simulink model "aircraft_6dof"  (R2025a)
settings: Solver=VariableStepAuto  StartTime=0.0  StopTime=sim_params.duration  FixedStep=0.01  RelTol=1e-8
values from neighbouring files (symbols this model uses):
  aero = evalin('base', 'aero')    [trim_solver.m]
  aircraft = evalin('base', 'aircraft')    [trim_solver.m]
  atmos = evalin('base', 'atmos')    [trim_solver.m]
  engine = evalin('base', 'engine')    [trim_solver.m]
undefined symbols (not defined in the file or in its folder): IC
libraries: aerolibasang x2, aerolibtransform2 x1, aerolibatmos2 x1
settings Model: Creator=lordf  LastModifiedBy=lordf
settings DataIOCC: ExternalInput=getinputstruct(op2)  InitialState=getstatestruct(op2)  LoadExternalInput=on  LoadInitialState=on

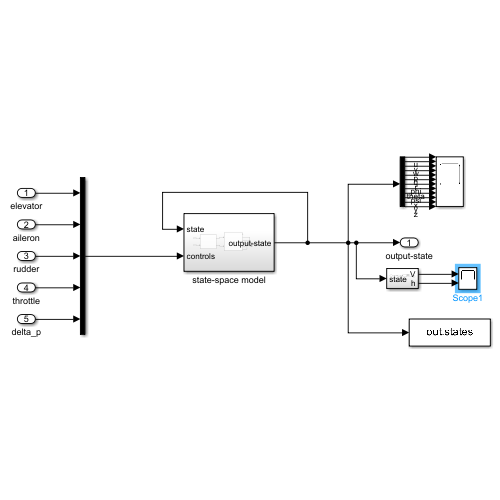
[thumbnail: Simulink's stored preview of the top-level diagram]
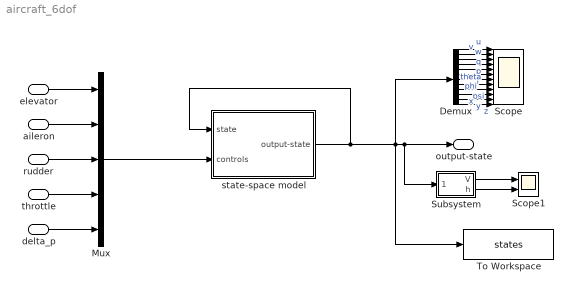
== system aircraft_6dof ==
  elevator : Inport
  aileron : Inport  Port=2
  rudder : Inport  Port=3
  throttle : Inport  Port=4
  delta_p : Inport  Port=5
  Demux : Demux  Outputs=12
  Mux : Mux  Inputs=5
  Scope : Scope  NumInputPorts=12
      settings: ActiveDisplayYMinimum=-1  ActiveDisplayYMaximum=1
  Scope1 : Scope  NumInputPorts=2
      settings: ActiveDisplayYMinimum=149.99795642842278  ActiveDisplayYMaximum=149.99795643262632
  Subsystem : Subsystem
  To Workspace : ToWorkspace  VariableName=states  SampleTime=-1
  state-space model : Subsystem
  output-state : Outport
  wires:
  state-space model/1(output-state) -> state-space model/1(state), Subsystem/1(state), output-state/1, Demux/1, To Workspace/1
  rudder/1 -> Mux/3
  aileron/1 -> Mux/2
  elevator/1 -> Mux/1
  throttle/1 -> Mux/4
  delta_p/1 -> Mux/5
  Mux/1 -> state-space model/2(controls)
  Demux/1 -> Scope/1  "u"
  Demux/2 -> Scope/2  "v"
  Demux/3 -> Scope/3  "w"
  Demux/4 -> Scope/4  "p"
  Demux/5 -> Scope/5  "q"
  Demux/6 -> Scope/6  "r"
  Demux/7 -> Scope/7  "phi"
  Demux/8 -> Scope/8  "theta"
  Demux/9 -> Scope/9  "psi"
  Demux/10 -> Scope/10  "x"
  Demux/11 -> Scope/11  "y"
  Demux/12 -> Scope/12  "z"
  Subsystem/2(h) -> Scope1/2
  Subsystem/1(V) -> Scope1/1

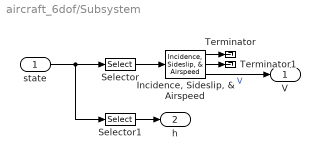
== system aircraft_6dof/Subsystem ==
  state : Inport
  "Incidence, Sideslip, & Airspeed" : aerolibasang/Incidence, Sideslip, & Airspeed
  Selector : Selector  InputPortWidth=12  IndexOptions=Index vector (dialog)  Indices=1:3  OutputSizes=1
  Selector1 : Selector  InputPortWidth=12  IndexOptions=Index vector (dialog)  Indices=12  OutputSizes=1
  Terminator : Terminator
  Terminator1 : Terminator
  V : Outport
  h : Outport  Port=2
  wires:
  Selector/1 -> "Incidence, Sideslip, & Airspeed"/1
  state/1 -> Selector1/1, Selector/1
  "Incidence, Sideslip, & Airspeed"/1 -> Terminator/1
  "Incidence, Sideslip, & Airspeed"/2 -> Terminator1/1
  "Incidence, Sideslip, & Airspeed"/3 -> V/1  "V"
  Selector1/1 -> h/1

== system aircraft_6dof/state-space model ==
  state : Inport
  controls : Inport  Port=2
  6DOF (Euler Angles) : EOM6DOFBodyEuler  xme_0=[IC.x IC.y IC.z]  Vm_0=[IC.u, IC.v, IC.w]  eul_0=[IC.phi IC.theta IC.psi]  pm_0=[IC.p IC.q IC.r]  mass_0=aircraft.mass  inertia=aircraft.I
  Forces and Moments : Subsystem
  Mux1 : Mux
  output-state : Outport
  wires:
  6DOF (Euler Angles)/3 -> Mux1/3  "attitude(earth)"
  6DOF (Euler Angles)/5 -> Mux1/1  "velocity(body)"
  Forces and Moments/2(M) -> 6DOF (Euler Angles)/2
  6DOF (Euler Angles)/2 -> Mux1/4  "Position(earth)"
  Forces and Moments/1(F) -> 6DOF (Euler Angles)/1
  6DOF (Euler Angles)/6 -> Mux1/2  "omega(body)"
  Mux1/1 -> output-state/1
  controls/1 -> Forces and Moments/2(controls)
  state/1 -> Forces and Moments/1(state)

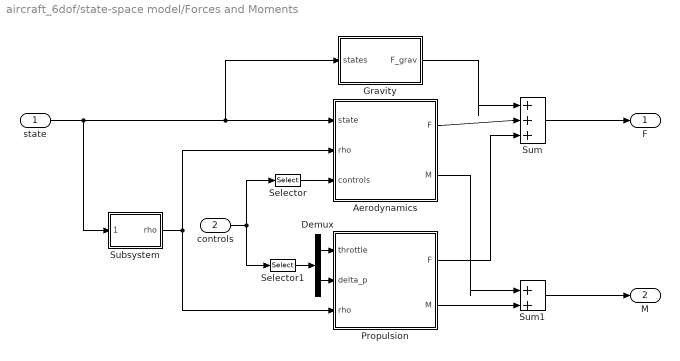
== system aircraft_6dof/state-space model/Forces and Moments ==
  state : Inport
  controls : Inport  Port=2
  Aerodynamics : Subsystem
  Demux : Demux  Outputs=2
  Gravity : Subsystem
  Propulsion : Subsystem
  Selector : Selector  InputPortWidth=5  IndexOptions=Index vector (dialog)  Indices=1:3  OutputSizes=1
  Selector1 : Selector  InputPortWidth=5  IndexOptions=Index vector (dialog)  Indices=4:5  OutputSizes=1
  Subsystem : Subsystem
  Sum : Sum  Inputs=|+++
  Sum1 : Sum  Inputs=|++
  F : Outport
  M : Outport  Port=2
  wires:
  Sum/1 -> F/1
  Aerodynamics/1(F) -> Sum/2
  Aerodynamics/2(M) -> Sum1/1
  Gravity/1(F_grav) -> Sum/1
  Sum1/1 -> M/1
  Demux/1 -> Propulsion/1(throttle)
  Demux/2 -> Propulsion/2(delta_p)
  Propulsion/1(F) -> Sum/3
  Propulsion/2(M) -> Sum1/2
  Subsystem/1(rho) -> Aerodynamics/2(rho), Propulsion/3(rho)
  Selector/1 -> Aerodynamics/3(controls)
  Selector1/1 -> Demux/1
  controls/1 -> Selector1/1, Selector/1
  state/1 -> Subsystem/1(states), Aerodynamics/1(state), Gravity/1(states)

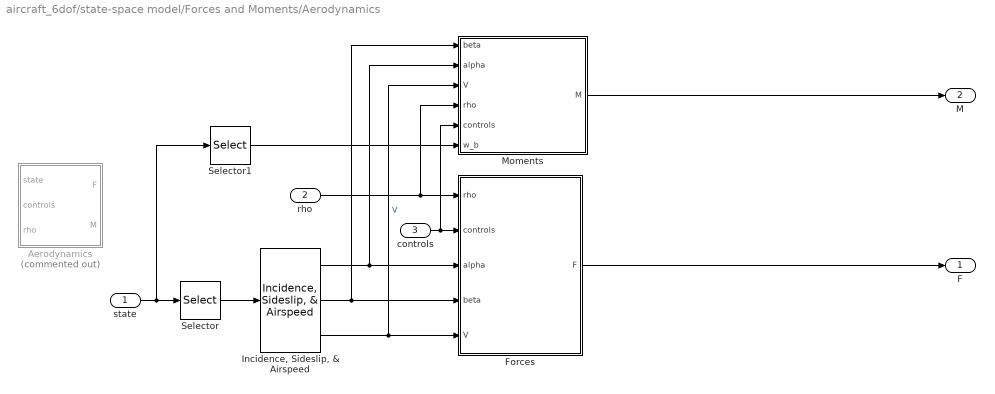
== system aircraft_6dof/state-space model/Forces and Moments/Aerodynamics ==
  state : Inport
  rho : Inport  Port=2
  controls : Inport  Port=3
  Aerodynamics : MATLAB Function  Commented=on  TreatAsAtomicUnit=on
  Forces : Subsystem
  "Incidence, Sideslip, & Airspeed" : aerolibasang/Incidence, Sideslip, & Airspeed
  Moments : Subsystem
  Selector : Selector  InputPortWidth=12  IndexOptions=Index vector (dialog)  Indices=1:3  OutputSizes=1
  Selector1 : Selector  InputPortWidth=12  IndexOptions=Index vector (dialog)  Indices=4:6  OutputSizes=1
  F : Outport
  M : Outport  Port=2
  wires:
  state/1 -> Selector/1, Selector1/1
  Moments/1(M) -> M/1
  Selector/1 -> "Incidence, Sideslip, & Airspeed"/1
  "Incidence, Sideslip, & Airspeed"/1 -> Forces/3(alpha), Moments/2(alpha)
  "Incidence, Sideslip, & Airspeed"/2 -> Forces/4(beta), Moments/1(beta)
  Forces/1(F) -> F/1
  "Incidence, Sideslip, & Airspeed"/3 -> Forces/5(V), Moments/3(V)  "V"
  rho/1 -> Forces/1(rho), Moments/4(rho)
  controls/1 -> Moments/5(controls), Forces/2(controls)
  Selector1/1 -> Moments/6(w_b)

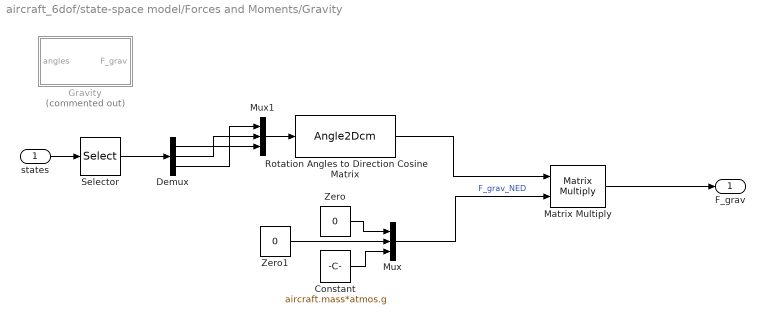
== system aircraft_6dof/state-space model/Forces and Moments/Gravity ==
  states : Inport
  Constant : Constant  Value=aircraft.mass*atmos.g
  Demux : Demux  Outputs=3
  Gravity : MATLAB Function  Commented=on  TreatAsAtomicUnit=on
  Matrix Multiply : Product  Multiplication=Matrix(*)
  Mux : Mux  Inputs=3
  Mux1 : Mux  Inputs=3
  Rotation Angles to Direction Cosine Matrix : Angle2Dcm
      settings: AttributesFormatString=Rotation Order: %<rotationOrder>
  Selector : Selector  InputPortWidth=12  IndexOptions=Index vector (dialog)  Indices=7:9  OutputSizes=1
  Zero : Constant  Value=0  OutDataTypeStr=Inherit: Inherit via back propagation
  Zero1 : Constant  Value=0  OutDataTypeStr=Inherit: Inherit via back propagation
  F_grav : Outport
  wires:
  Matrix Multiply/1 -> F_grav/1
  states/1 -> Selector/1
  Selector/1 -> Demux/1
  Zero/1 -> Mux/1
  Zero1/1 -> Mux/2
  Constant/1 -> Mux/3
  Mux/1 -> Matrix Multiply/2  "F_grav_NED"
  Demux/2 -> Mux1/2
  Demux/1 -> Mux1/3
  Demux/3 -> Mux1/1
  Mux1/1 -> Rotation Angles to Direction Cosine Matrix/1
  Rotation Angles to Direction Cosine Matrix/1 -> Matrix Multiply/1

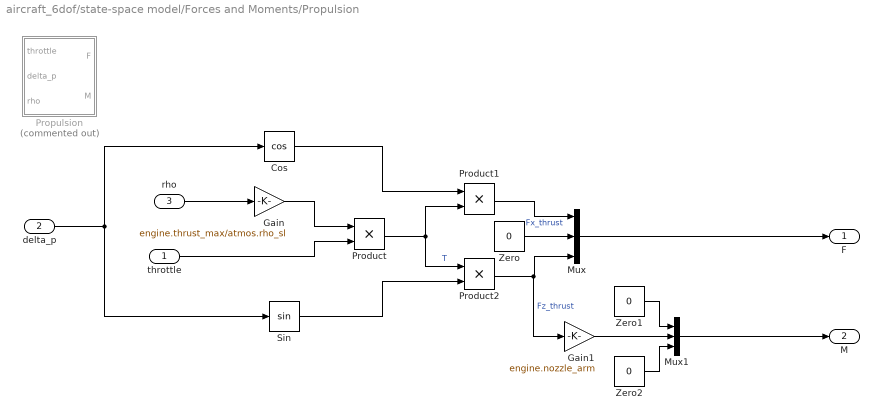
== system aircraft_6dof/state-space model/Forces and Moments/Propulsion ==
  throttle : Inport
  delta_p : Inport  Port=2
  rho : Inport  Port=3
  Cos : Trigonometry  Operator=cos
  Gain : Gain  Gain=engine.thrust_max/atmos.rho_sl
  Gain1 : Gain  Gain=engine.nozzle_arm
  Mux : Mux  Inputs=3
  Mux1 : Mux  Inputs=3
  Product : Product
  Product1 : Product
  Product2 : Product
  Propulsion : MATLAB Function  Commented=on  TreatAsAtomicUnit=on
  Sin : Trigonometry
  Zero : Constant  Value=0  OutDataTypeStr=Inherit: Inherit via back propagation
  Zero1 : Constant  Value=0  OutDataTypeStr=Inherit: Inherit via back propagation
  Zero2 : Constant  Value=0  OutDataTypeStr=Inherit: Inherit via back propagation
  F : Outport
  M : Outport  Port=2
  wires:
  Gain1/1 -> Mux1/2
  delta_p/1 -> Sin/1, Cos/1
  rho/1 -> Gain/1
  Mux/1 -> F/1
  throttle/1 -> Product/2
  Gain/1 -> Product/1
  Product/1 -> Product2/1, Product1/2  "T"
  Cos/1 -> Product1/1
  Sin/1 -> Product2/2
  Product1/1 -> Mux/1  "Fx_thrust"
  Product2/1 -> Gain1/1, Mux/3  "Fz_thrust"
  Zero/1 -> Mux/2
  Mux1/1 -> M/1
  Zero1/1 -> Mux1/1
  Zero2/1 -> Mux1/3

== system aircraft_6dof/state-space model/Forces and Moments/Subsystem ==
  states : Inport
  Gain : Gain  Gain=-1
  ISA Atmosphere Model : aerolibatmos2/ISA Atmosphere Model  useExtended=off  action=None  custom=off  viscosityOut=off  g=9.80665  gamma=1.4  R=287.0531  L=0.0065  h_trop=11000  h_strat=20000  rho0=1.225  P0=101325  T0=288.15  h0=0  S=110.4  Tref=273.15  muref=1.716e-5
  Selector : Selector  InputPortWidth=12  IndexOptions=Index vector (dialog)  Indices=12  OutputSizes=1
  rho : Outport
  wires:
  Selector/1 -> Gain/1
  Gain/1 -> ISA Atmosphere Model/1
  ISA Atmosphere Model/4 -> rho/1
  states/1 -> Selector/1

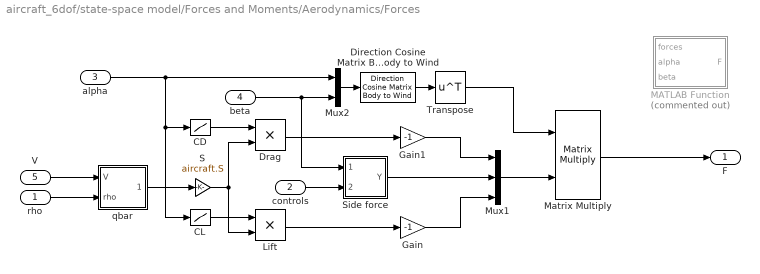
== system aircraft_6dof/state-space model/Forces and Moments/Aerodynamics/Forces ==
  rho : Inport
  controls : Inport  Port=2
  alpha : Inport  Port=3
  beta : Inport  Port=4
  V : Inport  Port=5
  CD : Lookup_n-D  NumberOfTableDimensions=1  BreakpointsForDimension1=aero.alpha_table  Table=aero.CD_data  InterpMethod=Cubic spline  ExtrapMethod=Clip  InternalRulePriority=Speed  RndMeth=Simplest
  CL : Lookup_n-D  NumberOfTableDimensions=1  BreakpointsForDimension1=aero.alpha_table  Table=aero.CL_data  InterpMethod=Cubic spline  ExtrapMethod=Clip  InternalRulePriority=Speed  RndMeth=Simplest
  Direction Cosine Matrix Body to Wind : aerolibtransform2/Direction Cosine Matrix Body to Wind
  Drag : Product
  Gain : Gain  Gain=-1
  Gain1 : Gain  Gain=-1
  Lift : Product
  MATLAB Function : MATLAB Function  Commented=on  TreatAsAtomicUnit=on
  Matrix Multiply : Product  Multiplication=Matrix(*)
  Mux1 : Mux  Inputs=3
  Mux2 : Mux  Inputs=2
  S : Gain  Gain=aircraft.S
  Side force : Subsystem
  Transpose : Math  Operator=transpose
  qbar : Subsystem
  F : Outport
  wires:
  beta/1 -> Side force/1(Beta), Mux2/2
  qbar/1(qbar) -> S/1
  Drag/1 -> Gain1/1
  Mux1/1 -> Matrix Multiply/2
  Lift/1 -> Gain/1
  Gain1/1 -> Mux1/1
  Matrix Multiply/1 -> F/1
  Gain/1 -> Mux1/3
  CL/1 -> Lift/1
  Side force/1(Y) -> Mux1/2
  alpha/1 -> Mux2/1, CD/1, CL/1
  controls/1 -> Side force/2(controls)
  V/1 -> qbar/1(V)
  rho/1 -> qbar/2(rho)
  Direction Cosine Matrix Body to Wind/1 -> Transpose/1
  Transpose/1 -> Matrix Multiply/1
  Mux2/1 -> Direction Cosine Matrix Body to Wind/1
  CD/1 -> Drag/1
  S/1 -> Drag/2, Lift/2

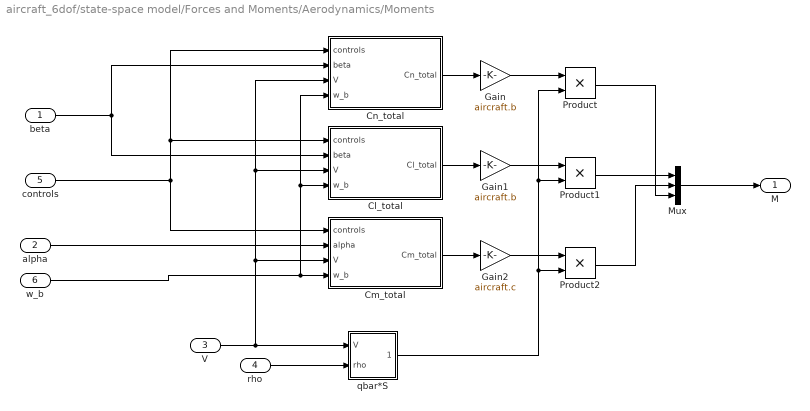
== system aircraft_6dof/state-space model/Forces and Moments/Aerodynamics/Moments ==
  beta : Inport
  alpha : Inport  Port=2
  V : Inport  Port=3
  rho : Inport  Port=4
  controls : Inport  Port=5
  w_b : Inport  Port=6
  Cl_total : Subsystem
  Cm_total : Subsystem
  Cn_total : Subsystem
  Gain : Gain  Gain=aircraft.b
  Gain1 : Gain  Gain=aircraft.b
  Gain2 : Gain  Gain=aircraft.c
  Mux : Mux  Inputs=3
  Product : Product
  Product1 : Product
  Product2 : Product
  qbar*S : Subsystem
  M : Outport
  wires:
  rho/1 -> qbar*S/2(rho)
  V/1 -> qbar*S/1(V), Cn_total/3(V), Cl_total/3(V), Cm_total/3(V)
  qbar*S/1(qbar*S) -> Product2/2, Product1/2, Product/2
  alpha/1 -> Cm_total/2(alpha)
  Cm_total/1(Cm_total) -> Gain2/1
  controls/1 -> Cn_total/1(controls), Cl_total/1(controls), Cm_total/1(controls)
  w_b/1 -> Cn_total/4(w_b), Cl_total/4(w_b), Cm_total/4(w_b)
  beta/1 -> Cn_total/2(beta), Cl_total/2(beta)
  Mux/1 -> M/1
  Cl_total/1(Cl_total) -> Gain1/1
  Cn_total/1(Cn_total) -> Gain/1
  Gain/1 -> Product/1
  Gain1/1 -> Product1/1
  Gain2/1 -> Product2/1
  Product1/1 -> Mux/1
  Product2/1 -> Mux/2
  Product/1 -> Mux/3

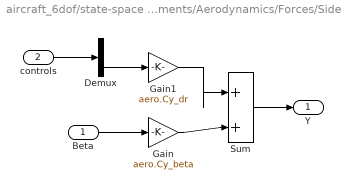
== system aircraft_6dof/state-space model/Forces and Moments/Aerodynamics/Forces/Side force ==
  Beta : Inport
  controls : Inport  Port=2
  Demux : Demux  Outputs=3
  Gain : Gain  Gain=aero.Cy_beta
  Gain1 : Gain  Gain=aero.Cy_dr
  Sum : Sum  Inputs=|++
  Y : Outport
  wires:
  Beta/1 -> Gain/1
  Gain/1 -> Sum/2
  Gain1/1 -> Sum/1
  Sum/1 -> Y/1
  controls/1 -> Demux/1
  Demux/3 -> Gain1/1

== system aircraft_6dof/state-space model/Forces and Moments/Aerodynamics/Forces/qbar ==
  V : Inport
  rho : Inport  Port=2
  Gain : Gain  Gain=0.5
  Math Function : Math  Operator=square
  Product : Product
  qbar : Outport
  wires:
  Math Function/1 -> Product/1
  rho/1 -> Gain/1
  Gain/1 -> Product/2
  Product/1 -> qbar/1
  V/1 -> Math Function/1

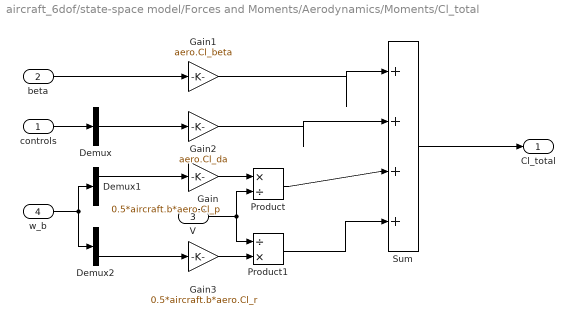
== system aircraft_6dof/state-space model/Forces and Moments/Aerodynamics/Moments/Cl_total ==
  controls : Inport
  beta : Inport  Port=2
  V : Inport  Port=3
  w_b : Inport  Port=4
  Demux : Demux  Outputs=3
  Demux1 : Demux  Outputs=3
  Demux2 : Demux  Outputs=3
  Gain : Gain  Gain=0.5*aircraft.b*aero.Cl_p
  Gain1 : Gain  Gain=aero.Cl_beta
  Gain2 : Gain  Gain=aero.Cl_da
  Gain3 : Gain  Gain=0.5*aircraft.b*aero.Cl_r
  Product : Product  Inputs=*/
  Product1 : Product  Inputs=/*
  Sum : Sum  Inputs=|++++
  Cl_total : Outport
  wires:
  Sum/1 -> Cl_total/1
  Product/1 -> Sum/3
  controls/1 -> Demux/1
  V/1 -> Product/2, Product1/1
  Gain/1 -> Product/1
  w_b/1 -> Demux1/1, Demux2/1
  Gain1/1 -> Sum/1
  beta/1 -> Gain1/1
  Demux/2 -> Gain2/1
  Demux1/1 -> Gain/1
  Product1/1 -> Sum/4
  Gain3/1 -> Product1/2
  Demux2/3 -> Gain3/1
  Gain2/1 -> Sum/2

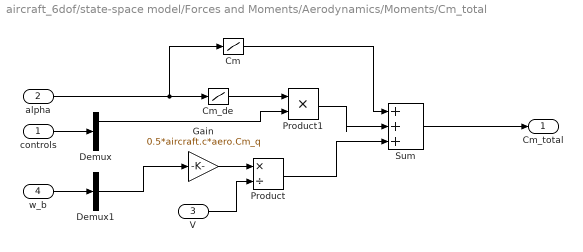
== system aircraft_6dof/state-space model/Forces and Moments/Aerodynamics/Moments/Cm_total ==
  controls : Inport
  alpha : Inport  Port=2
  V : Inport  Port=3
  w_b : Inport  Port=4
  Cm : Lookup_n-D  NumberOfTableDimensions=1  BreakpointsForDimension1=aero.alpha_table  Table=aero.Cm_data  InterpMethod=Cubic spline  ExtrapMethod=Clip  InternalRulePriority=Speed  RndMeth=Simplest
  Cm_de : Lookup_n-D  NumberOfTableDimensions=1  BreakpointsForDimension1=aero.alpha_table  Table=aero.Cm_de_data  InterpMethod=Cubic spline  ExtrapMethod=Clip  InternalRulePriority=Speed  RndMeth=Simplest
  Demux : Demux  Outputs=3
  Demux1 : Demux  Outputs=3
  Gain : Gain  Gain=0.5*aircraft.c*aero.Cm_q
  Product : Product  Inputs=*/
  Product1 : Product
  Sum : Sum  Inputs=|+++
  Cm_total : Outport
  wires:
  alpha/1 -> Cm_de/1, Cm/1
  Cm_de/1 -> Product1/1
  Cm/1 -> Sum/1
  w_b/1 -> Demux1/1
  Gain/1 -> Product/1
  V/1 -> Product/2
  controls/1 -> Demux/1
  Demux/1 -> Product1/2
  Product1/1 -> Sum/2
  Product/1 -> Sum/3
  Sum/1 -> Cm_total/1
  Demux1/2 -> Gain/1

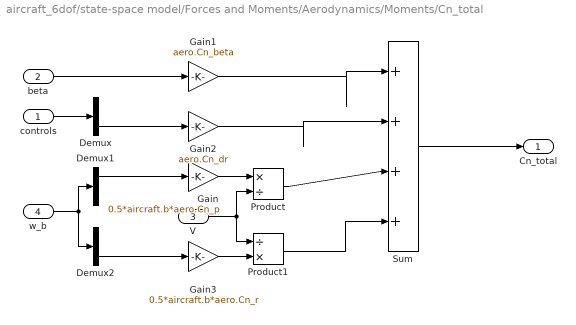
== system aircraft_6dof/state-space model/Forces and Moments/Aerodynamics/Moments/Cn_total ==
  controls : Inport
  beta : Inport  Port=2
  V : Inport  Port=3
  w_b : Inport  Port=4
  Demux : Demux  Outputs=3
  Demux1 : Demux  Outputs=3
  Demux2 : Demux  Outputs=3
  Gain : Gain  Gain=0.5*aircraft.b*aero.Cn_p
  Gain1 : Gain  Gain=aero.Cn_beta
  Gain2 : Gain  Gain=aero.Cn_dr
  Gain3 : Gain  Gain=0.5*aircraft.b*aero.Cn_r
  Product : Product  Inputs=*/
  Product1 : Product  Inputs=/*
  Sum : Sum  Inputs=|++++
  Cn_total : Outport
  wires:
  Gain2/1 -> Sum/2
  Demux2/3 -> Gain3/1
  Gain3/1 -> Product1/2
  Product1/1 -> Sum/4
  Demux1/1 -> Gain/1
  Demux/3 -> Gain2/1
  beta/1 -> Gain1/1
  Gain1/1 -> Sum/1
  w_b/1 -> Demux2/1, Demux1/1
  Gain/1 -> Product/1
  V/1 -> Product1/1, Product/2
  controls/1 -> Demux/1
  Product/1 -> Sum/3
  Sum/1 -> Cn_total/1

== system aircraft_6dof/state-space model/Forces and Moments/Aerodynamics/Moments/qbar*S ==
  V : Inport
  rho : Inport  Port=2
  Gain : Gain  Gain=0.5*aircraft.S
  Math Function : Math  Operator=square
  Product : Product
  qbar*S : Outport
  wires:
  V/1 -> Math Function/1
  Product/1 -> qbar*S/1
  Gain/1 -> Product/2
  rho/1 -> Gain/1
  Math Function/1 -> Product/1

== matlab function aircraft_6dof/state-space model/Forces and Moments/Propulsion/Propulsion ==
  data: throttle input; F output; delta_p input; rho input; M output; engine parameter
function [F,M] = propulsion(throttle, delta_p, rho, engine)
% Forces and moments due to nozzle in body frame

rho_sl = 1.225;           % kg/m^3


% Thrust magnitude (altitude corrected)
sigma = rho / rho_sl;
T = engine.thrust_max * throttle * sigma;

% Forces in body frame
Fx_thrust = T * cos(delta_p);
Fy_thrust = 0.0;
Fz_thrust = T * sin(delta_p);

% Moment about CG
Mx_thrust = 0.0;
My_thrust = Fz_thrust * engine.nozzle_arm;
Mz_thrust = 0.0;

% Output
F = [Fx_thrust; Fy_thrust; Fz_thrust];
M = [Mx_thrust; My_thrust; Mz_thrust];
end

== matlab function aircraft_6dof/state-space model/Forces and Moments/Aerodynamics/Aerodynamics ==
  data: state input; F output; controls input; rho input; M output; aero parameter; aircraft parameter
function [F,M]= aerodynamics(state, controls, rho, aero, aircraft)
% Aerodynamic forces and moments in body frame
% Unpack inputs
u = state(1); v = state(2); w = state(3);
p = state(4); q = state(5); r = state(6);
delta_e = controls(1); % elevator
delta_a = controls(2); % aileron
delta_r = controls(3); % rudder

% Flight parameters
V = sqrt(u^2+v^2+w^2);
if V<1e-6, V=1e-6; end
alpha = atan2(w,u);
beta = asin(v/V);

% Dynamic pressure
qbar = 0.5 * rho * V^2;

% Clamp alpha to table bounds
alpha_clamped = max(aero.alpha_min, min(alpha, aero.alpha_max));

% Interpolate aerodynamic coefficients using cubic spline
CL = interp1(aero.alpha_table, aero.CL_data, alpha_clamped, 'spline');
CD = interp1(aero.alpha_table, aero.CD_data, alpha_clamped, 'spline');
Cm = interp1(aero.alpha_table, aero.Cm_data, alpha_clamped, 'spline');
Cm_de = interp1(aero.alpha_table, aero.Cm_de_data, alpha_clamped, 'spline');

% Wind - frame forces
D = qbar * aircraft.S * CD; % Drag
L = qbar * aircraft.S * CL; % Lift
Y = qbar * aircraft.S * (aero.Cy_beta * beta + aero.Cy_dr * delta_r); % Side force

% Transform to body frame
ca = cos(alpha); sa = sin(alpha);
cb = cos(beta); sb = sin(beta);

% Aerodynamic forces
Fx_aero = -D * ca * cb - Y * sb + L * sa * cb;
Fy_aero = -D * ca * sb + Y * cb + L * sa * sb;
Fz_aero =  D * sa - L * ca;

% Aerodynamic moments
% Pitch Moment
Cm_total = Cm + aero.Cm_q*(q*aircraft.c/(2*V)) + Cm_de*delta_e;
My_aero = qbar * aircraft.S * aircraft.c * Cm_total;

% Roll Moment
Cl_beta_term = aero.Cl_beta * beta;
Cl_da_term   = aero.Cl_da * delta_a;
Cl_p_term    = aero.Cl_p * (p * aircraft.b / (2*V));
Cl_r_term    = aero.Cl_r * (r * aircraft.b / (2*V));
Mx_aero = qbar * aircraft.S * aircraft.b * (Cl_beta_term + Cl_da_term + Cl_p_term + Cl_r_term);

% Yaw Moment
Cn_beta_term = aero.Cn_beta * beta;
Cn_dr_term   = aero.Cn_dr * delta_r;
Cn_p_term    = aero.Cn_p * (p * aircraft.b / (2*V));
Cn_r_term    = aero.Cn_r * (r * aircraft.b / (2*V));
Mz_aero = qbar * aircraft.S * aircraft.b * (Cn_beta_term + Cn_dr_term + Cn_p_term + Cn_r_term);

% Output
F = [Fx_aero; Fy_aero; Fz_aero];
M = [Mx_aero; My_aero; Mz_aero];
end

== matlab function aircraft_6dof/state-space model/Forces and Moments/Gravity/Gravity ==
  data: angles input; F_grav output; atmos parameter; aircraft parameter
function F_grav = gravity(angles, atmos, aircraft)
    % Gravity
    g = atmos.g;
    m = aircraft.mass;
    phi = angles(1);
    theta = angles(2);
    psi = angles(3);
    F_grav_ned = [0; 0; m*g];

    cphi = cos(phi); sphi = sin(phi);
    cth = cos(theta); sth = sin(theta);
    cpsi = cos(psi); spsi = sin(psi);
    
    C_bn = [cth*cpsi, cth*spsi, -sth;
            sphi*sth*cpsi - cphi*spsi, sphi*sth*spsi + cphi*cpsi, sphi*cth;
            cphi*sth*cpsi + sphi*spsi, cphi*sth*spsi - sphi*cpsi, cphi*cth];
    
    F_grav = C_bn * F_grav_ned;

end

== matlab function aircraft_6dof/state-space model/Forces and Moments/Aerodynamics/Forces/MATLAB Function ==
  data: forces input; alpha input; F output; beta input
function F = fcn(forces,alpha,beta)
    % Transform to body frame
    ca = cos(alpha); sa = sin(alpha);
    cb = cos(beta);  sb = sin(beta);
    D = forces(1);
    Y = forces(2);
    L = forces(3);
    
    Fx_aero = -D * ca * cb - Y * sb + L * sa * cb;
    Fy_aero = -D * ca * sb + Y * cb + L * sa * sb;
    Fz_aero =  D * sa - L * ca;

    F = [Fx_aero;Fy_aero;Fz_aero];
